simulink model "topicsPlot"  (R2020b)
settings: Solver=FixedStepAuto  StartTime=52.0  StopTime=52.0+125.0  FixedStep=0.1  RelTol=1e-3
model workspace (MAT data in the model file):
  Logfile_Data_Object = robotics.ros.BagSelection
  Logfile_Data_Object.FilePath = '/media/fmccastro/My_Passport/Universidade/IST_repositorio_pessoal/5_ano_2_sem/Tese_RoverNavigation_root/Tese_RoverNavigation/ROS_workspaces/wsPy3/src/pioneer3at_control/bagfiles/subset.bag'
  Logfile_Data_Object.StartTime = 61.124
  Logfile_Data_Object.EndTime = 354.332
  Logfile_Data_Object.NumMessages = 780848
  Logfile_Data_Object.AvailableTopics = table
  Logfile_Data_Object.AvailableTopics.data{1} = [1094; 1094; 1094; 1094; 1094; 241225; 246357; 1094; 286702]
  Logfile_Data_Object.AvailableTopics.data{2} = categorical
  Logfile_Data_Object.AvailableTopics.data{2}.categoryNames = {'geometry_msgs/Twist'; 'pioneer3at_control/pose3D'; 'std_msgs/Float64'; 'std_msgs/Float64MultiArray'; 'std_msgs/Int32'}
  Logfile_Data_Object.AvailableTopics.data{2}.codes = [3; 1; 4; 4; 5; 3; 4; 3; 2]
  Logfile_Data_Object.AvailableTopics.data{3}{1} = ''
  Logfile_Data_Object.AvailableTopics.data{3}{2} = '  double X
    |   double Y
    |   double Z
    | geometry_msgs/Vector3 Angular
    |   double X
    |   double Y
    |   double Z
    | '
  Logfile_Data_Object.AvailableTopics.data{3}{3} = '  std_msgs/MultiArrayDimension[] Dim
    |     char Label
    |     uint32 Size
    |     uint32 Stride
    |   uint32 DataOffset
    | double[] Data
    | '
  Logfile_Data_Object.AvailableTopics.data{3}{4} = '  std_msgs/MultiArrayDimension[] Dim
    |     char Label
    |     uint32 Size
    |     uint32 Stride
    |   uint32 DataOffset
    | double[] Data
    | '
  Logfile_Data_Object.AvailableTopics.data{3}{5} = ''
  Logfile_Data_Object.AvailableTopics.data{3}{6} = ''
  Logfile_Data_Object.AvailableTopics.data{3}{7} = '  std_msgs/MultiArrayDimension[] Dim
    |     char Label
    |     uint32 Size
    |     uint32 Stride
    |   uint32 DataOffset
    | double[] Data
    | '
  Logfile_Data_Object.AvailableTopics.data{3}{8} = ''
  Logfile_Data_Object.AvailableTopics.data{3}{9} = 'single Y
    | single Z
    | single Roll
    | single Pitch
    | single Yaw
    | '
  Logfile_Data_Object.AvailableTopics.ndims = 2
  Logfile_Data_Object.AvailableTopics.nrows = 9
  Logfile_Data_Object.AvailableTopics.rownames = {'/pioneer3at/clock'; '/pioneer3at/cmd_vel'; '/pioneer3at/currentRef'; '/pioneer3at/currentSol'; '/pioneer3at/currentStep'; '/pioneer3at/distance'; '/pioneer3at/error'; '/pioneer3at/optTime'; '/pioneer3at/robotPose'}
  Logfile_Data_Object.AvailableTopics.nvars = 3
  Logfile_Data_Object.AvailableTopics.varnames = {'NumMessages', 'MessageType', 'MessageDefinition'}
  Logfile_Data_Object.AvailableTopics.props.useVariableNamesOriginal = 0
  Logfile_Data_Object.AvailableTopics.props.useDimensionNamesOriginal = 0
  Logfile_Data_Object.AvailableTopics.props.CustomProps = struct()
  Logfile_Data_Object.AvailableTopics.props.VariableCustomProps = struct()
  Logfile_Data_Object.AvailableTopics.props.versionSavedFrom = 4
  Logfile_Data_Object.AvailableTopics.props.minCompatibleVersion = 1
  Logfile_Data_Object.AvailableTopics.props.incompatibilityMsg = ''
  Logfile_Data_Object.AvailableTopics.props.VersionSavedFrom = 4
  Logfile_Data_Object.AvailableTopics.props.Description = ''
  Logfile_Data_Object.AvailableTopics.props.VariableNamesOriginal = {}
  Logfile_Data_Object.AvailableTopics.props.DimensionNames = {'Row', 'Variables'}
  Logfile_Data_Object.AvailableTopics.props.DimensionNamesOriginal = {}
  Logfile_Data_Object.AvailableTopics.props.UserData = []
  Logfile_Data_Object.AvailableTopics.props.VariableDescriptions = {}
  Logfile_Data_Object.AvailableTopics.props.VariableUnits = {}
  Logfile_Data_Object.AvailableTopics.props.VariableContinuity = {}
  Logfile_Data_Object.MessageList = table
  Logfile_Data_Object.MessageList.data{1} = [61.124 61.125 61.126 61.129 61.129 61.131 61.131 61.131 61.132 61.134 61.136 61.139 ... (780848 elements, 780848x1)]
  Logfile_Data_Object.MessageList.data{2} = categorical
  Logfile_Data_Object.MessageList.data{2}.categoryNames = {'/pioneer3at/clock'; '/pioneer3at/cmd_vel'; '/pioneer3at/currentRef'; '/pioneer3at/currentSol'; '/pioneer3at/currentStep'; '/pioneer3at/distance'; '/pioneer3at/error'; '/pioneer3at/optTime'; '/pioneer3at/robotPose'}
  Logfile_Data_Object.MessageList.data{2}.codes = [9 9 9 9 9 9 9 9 9 9 9 9 ... (780848 elements, 780848x1)]
  Logfile_Data_Object.MessageList.data{3} = categorical
  Logfile_Data_Object.MessageList.data{3}.categoryNames = {'std_msgs/Float64'; 'geometry_msgs/Twist'; 'std_msgs/Float64MultiArray'; 'std_msgs/Int32'; 'pioneer3at_control/pose3D'}
  Logfile_Data_Object.MessageList.data{3}.codes = [5 5 5 5 5 5 5 5 5 5 5 5 ... (780848 elements, 780848x1)]
  Logfile_Data_Object.MessageList.data{4} = [4466 4536 4606 4676 4746 4816 4886 4956 5026 5096 5166 5236 ... (780848 elements, 780848x1)]
  Logfile_Data_Object.MessageList.ndims = 2
  Logfile_Data_Object.MessageList.nrows = 780848
  Logfile_Data_Object.MessageList.nvars = 4
  Logfile_Data_Object.MessageList.varnames = {'Time', 'Topic', 'MessageType', 'FileOffset'}
  Logfile_Data_Object.MessageList.props.useVariableNamesOriginal = 0
  Logfile_Data_Object.MessageList.props.useDimensionNamesOriginal = 0
  Logfile_Data_Object.MessageList.props.CustomProps = struct()
  Logfile_Data_Object.MessageList.props.VariableCustomProps = struct()
  Logfile_Data_Object.MessageList.props.versionSavedFrom = 4
  Logfile_Data_Object.MessageList.props.minCompatibleVersion = 1
  Logfile_Data_Object.MessageList.props.incompatibilityMsg = ''
  Logfile_Data_Object.MessageList.props.VersionSavedFrom = 4
  Logfile_Data_Object.MessageList.props.Description = ''
  Logfile_Data_Object.MessageList.props.VariableNamesOriginal = {}
  Logfile_Data_Object.MessageList.props.DimensionNames = {'Row', 'Variables'}
  Logfile_Data_Object.MessageList.props.DimensionNamesOriginal = {}
  Logfile_Data_Object.MessageList.props.UserData = []
  Logfile_Data_Object.MessageList.props.VariableDescriptions = {}
  Logfile_Data_Object.MessageList.props.VariableUnits = {}
  Logfile_Data_Object.MessageList.props.VariableContinuity = {}
  Logfile_Data_Object.TopicTypeMap = containers.Map
  Logfile_Data_Object.TopicTypeMap.serialization.keys = {'/pioneer3at/clock', '/pioneer3at/cmd_vel', '/pioneer3at/currentRef', '/pioneer3at/currentSol', '/pioneer3at/currentStep', '/pioneer3at/distance', '/pioneer3at/error', '/pioneer3at/optTime', '/pioneer3at/robotPose'}
  Logfile_Data_Object.TopicTypeMap.serialization.values = {'std_msgs/Float64', 'geometry_msgs/Twist', 'std_msgs/Float64MultiArray', 'std_msgs/Float64MultiArray', 'std_msgs/Int32', 'std_msgs/Float64', 'std_msgs/Float64MultiArray', 'std_msgs/Float64', 'pioneer3at_control/pose3D'}
  Logfile_Data_Object.TopicTypeMap.serialization.uniformity = 1
  Logfile_Data_Object.TopicTypeMap.serialization.keyType = 'char'
  Logfile_Data_Object.TopicTypeMap.serialization.valueType = 'char'
  Logfile_Data_Object.TopicDefinitionMap = containers.Map
  Logfile_Data_Object.TopicDefinitionMap.serialization.keys = {'/pioneer3at/clock', '/pioneer3at/cmd_vel', '/pioneer3at/currentRef', '/pioneer3at/currentSol', '/pioneer3at/currentStep', '/pioneer3at/distance', '/pioneer3at/error', '/pioneer3at/optTime', '/pioneer3at/robotPose'}
  Logfile_Data_Object.TopicDefinitionMap.serialization.values{1} = ''
  Logfile_Data_Object.TopicDefinitionMap.serialization.values{2} = '  double X
    |   double Y
    |   double Z
    | geometry_msgs/Vector3 Angular
    |   double X
    |   double Y
    |   double Z
    | '
  Logfile_Data_Object.TopicDefinitionMap.serialization.values{3} = '  std_msgs/MultiArrayDimension[] Dim
    |     char Label
    |     uint32 Size
    |     uint32 Stride
    |   uint32 DataOffset
    | double[] Data
    | '
  Logfile_Data_Object.TopicDefinitionMap.serialization.values{4} = '  std_msgs/MultiArrayDimension[] Dim
    |     char Label
    |     uint32 Size
    |     uint32 Stride
    |   uint32 DataOffset
    | double[] Data
    | '
  Logfile_Data_Object.TopicDefinitionMap.serialization.values{5} = ''
  Logfile_Data_Object.TopicDefinitionMap.serialization.values{6} = ''
  Logfile_Data_Object.TopicDefinitionMap.serialization.values{7} = '  std_msgs/MultiArrayDimension[] Dim
    |     char Label
    |     uint32 Size
    |     uint32 Stride
    |   uint32 DataOffset
    | double[] Data
    | '
  Logfile_Data_Object.TopicDefinitionMap.serialization.values{8} = ''
  Logfile_Data_Object.TopicDefinitionMap.serialization.values{9} = 'single Y
    | single Z
    | single Roll
    | single Pitch
    | single Yaw
    | '
  Logfile_Data_Object.TopicDefinitionMap.serialization.uniformity = 1
  Logfile_Data_Object.TopicDefinitionMap.serialization.keyType = 'char'
  Logfile_Data_Object.TopicDefinitionMap.serialization.valueType = 'char'
  Logfile_Data_Object.messageTypeMap = containers.Map
  Logfile_Data_Object.messageTypeMap.serialization.keys = {}
  Logfile_Data_Object.messageTypeMap.serialization.values = {}
  Logfile_Data_Object.messageTypeMap.serialization.uniformity = 0
  Logfile_Data_Object.messageTypeMap.serialization.keyType = 'char'
  Logfile_Data_Object.messageTypeMap.serialization.valueType = 'any'
  Logfile_Data_Object.Parser = robotics.ros.internal.tf.TransformationTreeParser
  Logfile_Path = '/media/fmccastro/My_Passport/Universidade/IST_repositorio_pessoal/5_ano_2_sem/Tese_RoverNavigation_root/Tese_RoverNavigation/ROS_workspaces/wsPy3/src/pioneer3at_control/bagfiles/subset.bag'
  Logfile_Playback_Duration = nan
  Logfile_Playback_Offset = nan
undefined symbols (not defined in the file or in its folder): pioneer3at_control, pose3D
libraries: robotlib x3
settings Model: Creator=fmccastro  LastModifiedBy=fmccastro

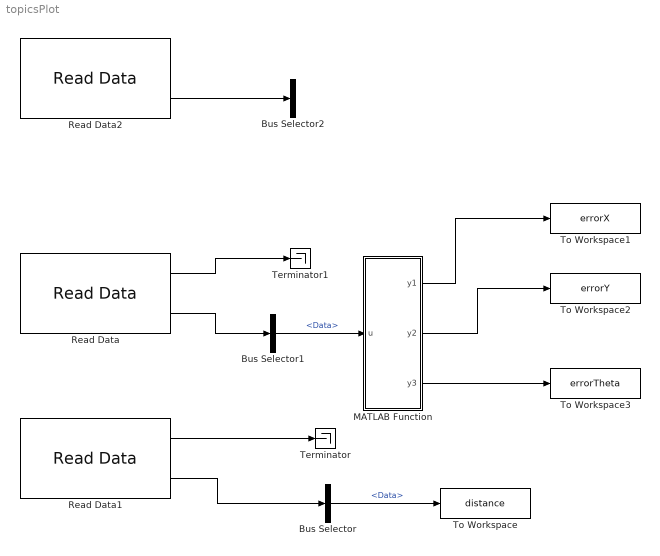
== system topicsPlot ==
  Bus Selector : BusSelector  OutputSignals=Data
  Bus Selector1 : BusSelector  OutputSignals=Data
  Bus Selector2 : BusSelector  OutputSignals=Data
  MATLAB Function : MATLAB Function  TreatAsAtomicUnit=on
  Read Data : robotlib/Read Data  topic=/pioneer3at/error  sampleTime=-1  logfileType=rosbag  modelName=topicsPlot  msgType=std_msgs/Float64MultiArray
      settings: SourceProductBaseCode=RR
  Read Data1 : robotlib/Read Data  topic=/pioneer3at/distance  sampleTime=-1  logfileType=rosbag  modelName=topicsPlot  msgType=std_msgs/Float64
      settings: SourceProductBaseCode=RR
  Read Data2 : robotlib/Read Data  topic=/pioneer3at/robotPose  sampleTime=-1  logfileType=rosbag  modelName=topicsPlot  msgType=pioneer3at_control/pose3D
      settings: SourceProductBaseCode=RR
  Terminator : Terminator
  Terminator1 : Terminator
  To Workspace : ToWorkspace  VariableName=distance  SaveFormat=Timeseries  SampleTime=-1
  To Workspace1 : ToWorkspace  VariableName=errorX  SaveFormat=Timeseries  SampleTime=-1
  To Workspace2 : ToWorkspace  VariableName=errorY  SaveFormat=Timeseries  SampleTime=-1
  To Workspace3 : ToWorkspace  VariableName=errorTheta  SaveFormat=Timeseries  SampleTime=-1
  wires:
  Bus Selector1/1 -> MATLAB Function/1(u)  "<Data>"
  Read Data/2 -> Bus Selector1/1
  Read Data1/2 -> Bus Selector/1
  Read Data1/1 -> Terminator/1
  Read Data/1 -> Terminator1/1
  Bus Selector/1 -> To Workspace/1  "<Data>"
  MATLAB Function/1(y1) -> To Workspace1/1
  MATLAB Function/2(y2) -> To Workspace2/1
  MATLAB Function/3(y3) -> To Workspace3/1
  Read Data2/2 -> Bus Selector2/1

== matlab function topicsPlot/MATLAB Function ==
  data: u input; y1 output; y2 output; y3 output
function [y1, y2, y3] = fcn(u)

y1 = u(1);
y2 = u(2);
y3 = u(3);
